simulink model "top_level"  (R2024b)
settings: Solver=VariableStepAuto  StartTime=0.0  StopTime=30  RelTol=1e-3
PreLoadFcn:
  | init_params
InitFcn:
  | mdlFile  = get_param(bdroot,'FileName');
  | mdlDir   = fileparts(mdlFile);
  | projRoot = fileparts(mdlDir);
  | addpath(genpath(projRoot));
  | run(fullfile(projRoot,'scripts','init_params.m'));
undefined symbols (not defined in the file): A_EGT, a_thrust, B_EGT, b_Neq, dWf_dn_max, dWf_up_max, EGT_idle, EGT_max, f_tbl, I_N_max, I_N_min, K_aw, k_Neq, Ki_N, Ki_T, Kp_N, Kp_T, N_idle, N_init, N_max_ref, T_max, tau_EGT, tau_N, throttle_bp, Wf_idle, Wf_max, Wf_min
libraries: simulink x1, simulink_extras x1
settings Model: Creator=rodog  LastModifiedBy=rodog
settings DebuggingCC: InheritedTsInSrcMsg=none

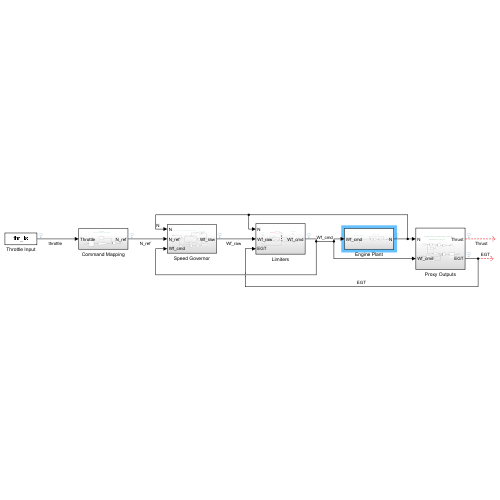
[thumbnail: Simulink's stored preview of the top-level diagram]
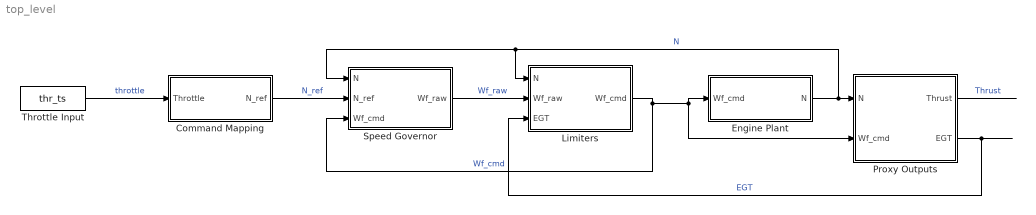
== system top_level ==
  Command Mapping : Subsystem
  Engine Plant : Subsystem
  Limiters : Subsystem
  Proxy Outputs : Subsystem
  Speed Governor : Subsystem
  Throttle Input : FromWorkspace  VariableName=thr_ts  SampleTime=-1  Interpolate=off  OutputAfterFinalValue=Holding final value
  wires:
  Throttle Input/1 -> Command Mapping/1(Throttle)  "throttle"
  Speed Governor/1(Wf_raw) -> Limiters/2(Wf_raw)  "Wf_raw"
  Command Mapping/1(N_ref) -> Speed Governor/2(N_ref)  "N_ref"
  Limiters/1(Wf_cmd) -> Proxy Outputs/2(Wf_cmd), Engine Plant/1(Wf_cmd), Speed Governor/3(Wf_cmd)  "Wf_cmd"
  Engine Plant/1(N) -> Proxy Outputs/1(N), Limiters/1(N), Speed Governor/1(N)  "N"
  Proxy Outputs/1(Thrust) -> ?  "Thrust"
  Proxy Outputs/2(EGT) -> Limiters/3(EGT)  "EGT"

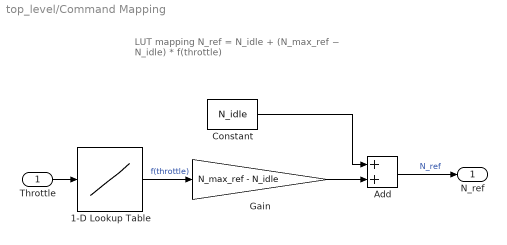
== system top_level/Command Mapping ==
  note: LUT mapping
      | N_ref ​= N_idle​ + (N_max_ref ​− N_idle​) * f(throttle)
  Throttle : Inport
  1-D Lookup Table : Lookup_n-D  NumberOfTableDimensions=1  BreakpointsForDimension1=throttle_bp  Table=f_tbl  ExtrapMethod=Clip  InternalRulePriority=Speed  RndMeth=Simplest
  Add : Sum
  Constant : Constant  Value=N_idle
  Gain : Gain  Gain=N_max_ref - N_idle
  N_ref : Outport
  wires:
  Throttle/1 -> 1-D Lookup Table/1
  Add/1 -> N_ref/1  "N_ref"
  1-D Lookup Table/1 -> Gain/1  "f(throttle)"
  Gain/1 -> Add/2
  Constant/1 -> Add/1

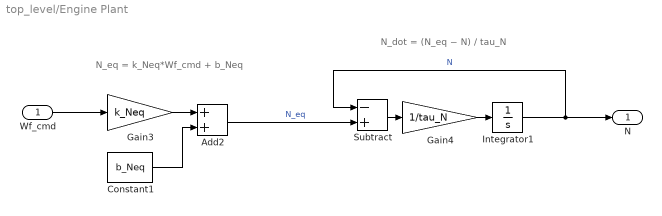
== system top_level/Engine Plant ==
  note: N_dot = (N_e​q − N) / tau_N​
  note: N_eq = k_Neq*Wf_cmd + b_Neq
  Wf_cmd : Inport
  Add2 : Sum
  Constant1 : Constant  Value=b_Neq
  Gain3 : Gain  Gain=k_Neq
  Gain4 : Gain  Gain=1/tau_N
  Integrator1 : Integrator  InitialCondition=N_init
  Subtract : Sum  Inputs=-+
  N : Outport
  wires:
  Gain4/1 -> Integrator1/1
  Add2/1 -> Subtract/2  "N_eq"
  Gain3/1 -> Add2/1
  Constant1/1 -> Add2/2
  Subtract/1 -> Gain4/1
  Wf_cmd/1 -> Gain3/1
  Integrator1/1 -> Subtract/1, N/1  "N"

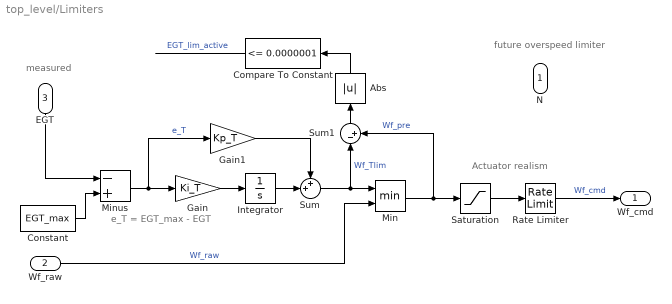
== system top_level/Limiters ==
  note: future overspeed limiter
  note: measured
  note: e_T = EGT_max - EGT
  note: Actuator realism
  N : Inport
  Wf_raw : Inport  Port=2
  EGT : Inport  Port=3
  Abs : Abs  SaturateOnIntegerOverflow=off
  Compare To Constant : simulink/Logic and Bit Operations/Compare To Constant  relop=<=  const=0.0000001  OutDataTypeStr=boolean
  Constant : Constant  Value=EGT_max
  Gain : Gain  Gain=Ki_T
  Gain1 : Gain  Gain=Kp_T
  Integrator : Integrator  InitialCondition=Wf_max  LimitOutput=on  UpperSaturationLimit=Wf_max  LowerSaturationLimit=Wf_min
  Min : MinMax  Inputs=2
  Minus : Sum  Inputs=-+
  Rate Limiter : RateLimiter  RisingSlewLimit=dWf_up_max  FallingSlewLimit=-dWf_dn_max  SampleTimeMode=inherited  InitialCondition=Wf_idle
  Saturation : Saturate  UpperLimit=Wf_max  LowerLimit=Wf_min
  Sum : Sum  Inputs=++|
  Sum1 : Sum  Inputs=|-+
  Wf_cmd : Outport
  wires:
  Saturation/1 -> Rate Limiter/1
  Rate Limiter/1 -> Wf_cmd/1  "Wf_cmd"
  Min/1 -> Sum1/2, Saturation/1  "Wf_pre"
  Wf_raw/1 -> Min/2  "Wf_raw"
  EGT/1 -> Minus/1
  Minus/1 -> Gain1/1, Gain/1  "e_T"
  Gain/1 -> Integrator/1
  Sum/1 -> Sum1/1, Min/1  "Wf_Tlim"
  Constant/1 -> Minus/2
  Integrator/1 -> Sum/2
  Gain1/1 -> Sum/1
  Sum1/1 -> Abs/1
  Compare To Constant/1 -> ?  "EGT_lim_active"
  Abs/1 -> Compare To Constant/1

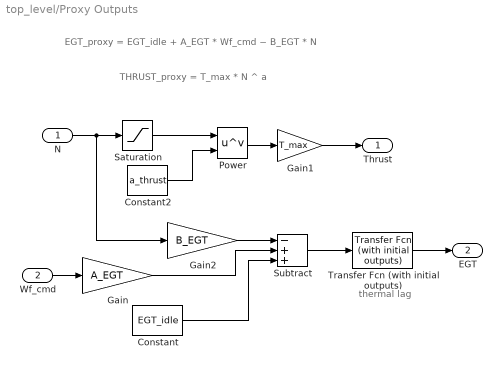
== system top_level/Proxy Outputs ==
  note: thermal lag
  note: THRUST_proxy = T_max * N ^ a
  note: EGT_proxy = EGT_idle + A_EGT * Wf_cmd − B_EGT * N
  N : Inport
  Wf_cmd : Inport  Port=2
  Constant : Constant  Value=EGT_idle
  Constant2 : Constant  Value=a_thrust
  Gain : Gain  Gain=A_EGT
  Gain1 : Gain  Gain=T_max
  Gain2 : Gain  Gain=B_EGT
  Power : Math  Operator=pow
  Saturation : Saturate  UpperLimit=1.2  LowerLimit=0
  Subtract : Sum  Inputs=-++
  Transfer Fcn (with initial outputs) : simulink_extras/Additional Linear/Transfer Fcn (with initial outputs)  N=[1]  D="[tau_EGT  1]"  Y0=EGT_init  U0=0
  Thrust : Outport
  EGT : Outport  Port=2
  wires:
  N/1 -> Gain2/1, Saturation/1
  Wf_cmd/1 -> Gain/1
  Saturation/1 -> Power/1
  Subtract/1 -> Transfer Fcn (with initial outputs)/1
  Constant2/1 -> Power/2
  Power/1 -> Gain1/1
  Gain1/1 -> Thrust/1
  Constant/1 -> Subtract/3
  Gain/1 -> Subtract/2
  Gain2/1 -> Subtract/1
  Transfer Fcn (with initial outputs)/1 -> EGT/1

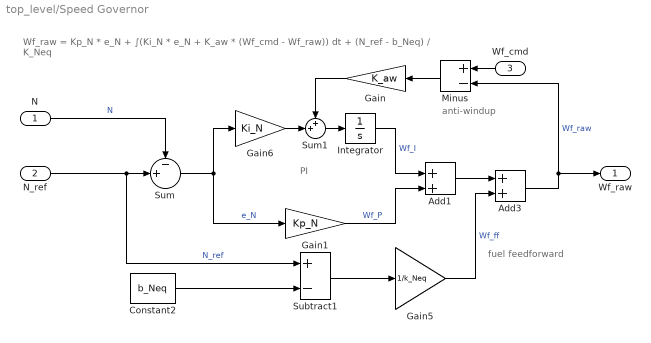
== system top_level/Speed Governor ==
  note: Wf_raw = Kp_N * e_N + ∫(Ki_N * e_N + K_aw * (Wf_cmd - Wf_raw)) dt + (N_ref - b_Neq) / K_Neq
  note: PI
  note: fuel feedforward
  note: anti-windup
  N : Inport
  N_ref : Inport  Port=2
  Wf_cmd : Inport  Port=3
  Add1 : Sum  Inputs=+|+
  Add3 : Sum
  Constant2 : Constant  Value=b_Neq
  Gain : Gain  Gain=K_aw
  Gain1 : Gain  Gain=Kp_N
  Gain5 : Gain  Gain=1/k_Neq
  Gain6 : Gain  Gain=Ki_N
  Integrator : Integrator  LimitOutput=on  UpperSaturationLimit=I_N_max  LowerSaturationLimit=I_N_min
  Minus : Sum  Inputs=+-
  Subtract1 : Sum  Inputs=+-
  Sum : Sum  Inputs=-+|
  Sum1 : Sum  Inputs=++|
  Wf_raw : Outport
  wires:
  N_ref/1 -> Subtract1/1, Sum/2  "N_ref"
  N/1 -> Sum/1  "N"
  Integrator/1 -> Add1/1  "Wf_I"
  Subtract1/1 -> Gain5/1
  Constant2/1 -> Subtract1/2
  Sum/1 -> Gain6/1, Gain1/1  "e_N"
  Gain1/1 -> Add1/2  "Wf_P"
  Add1/1 -> Add3/1
  Gain5/1 -> Add3/2  "Wf_ff"
  Add3/1 -> Minus/2, Wf_raw/1  "Wf_raw"
  Wf_cmd/1 -> Minus/1
  Minus/1 -> Gain/1
  Gain6/1 -> Sum1/2
  Sum1/1 -> Integrator/1
  Gain/1 -> Sum1/1
